simulink model "TransmissionController"  (R2023b)
settings: configuration reference "VehicleFixed10ms" (kept outside this file)
StartFcn:
  | %tic
StopFcn:
  | %toc
libraries: autolibtranscontrolscommon x1
settings Model: DataDictionary=VirtualVehicleTemplate.sldd  ModifiedByFormat=The MathWorks, Inc.  Creator=The MathWorks, Inc.  LastModifiedBy=The MathWorks, Inc.
settings ConfigSetRef: SourceName=VehicleFixed10ms

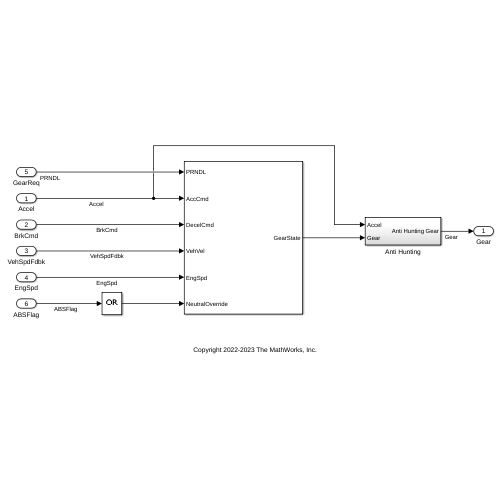
[thumbnail: Simulink's stored preview of the top-level diagram]
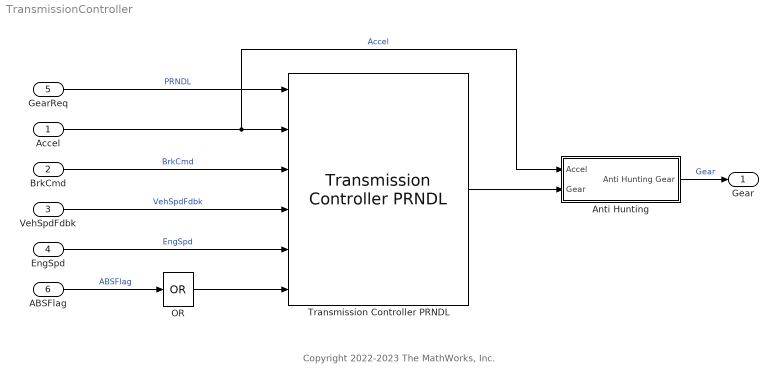
== system TransmissionController ==
  note: Copyright 2022-2023 The MathWorks, Inc.
  Accel : Inport  OutDataTypeStr=double  PortDimensions=1
  BrkCmd : Inport  Port=2  OutDataTypeStr=double  PortDimensions=1
  VehSpdFdbk : Inport  Port=3  OutDataTypeStr=double  Unit=m/s  PortDimensions=1
  EngSpd : Inport  Port=4  OutDataTypeStr=double  Unit=rad/s  PortDimensions=1
  GearReq : Inport  Port=5  OutDataTypeStr=double  PortDimensions=1
  ABSFlag : Inport  Port=6  OutDataTypeStr=boolean  PortDimensions=4
  Anti Hunting : Subsystem
  OR : Logic  Operator=OR  Inputs=1  AllPortsSameDT=off  OutDataTypeStr=boolean
  Transmission Controller PRNDL : autolibtranscontrolscommon/Transmission Controller PRNDL  DriveMode=off  GearInit=CtrlTcuInitGear  LugSpd=CtrlTcuLugSpd  MinUpSpd=CtrlTcuMinUpSpd  tClutchUp=CtrlTcuTmUpSh  tClutchDn=CtrlTcuTmDnSh  tPark=120  VelUnit=km/hr  UpShSpd=CtrlTcuUpShSpd  UpLdBpt=CtrlTcuUpLdBpt  UpShBpt=1:7  UpPtBpt=[1 2]  DnShfSpd=CtrlTcuDnShSpd  DnShSpd=CtrlTcuDnShSpd  DnLdBpt=CtrlTcuDnLdBpt  DnShBpt=2:8  DnPtBpt=[1 2]  POFS=zeros(4,1)  GOFS=zeros(1,7)  Ngears=8  aMode=6
  Gear : Outport  OutDataTypeStr=double  PortDimensions=1  VectorParamsAs1DForOutWhenUnconnected=off
  wires:
  ABSFlag/1 -> OR/1  "ABSFlag"
  Anti Hunting/1(Anti Hunting Gear) -> Gear/1  "Gear"
  GearReq/1 -> Transmission Controller PRNDL/1  "PRNDL"
  Accel/1 -> Anti Hunting/1(Accel), Transmission Controller PRNDL/2  "Accel"
  BrkCmd/1 -> Transmission Controller PRNDL/3  "BrkCmd"
  EngSpd/1 -> Transmission Controller PRNDL/5  "EngSpd"
  VehSpdFdbk/1 -> Transmission Controller PRNDL/4  "VehSpdFdbk"
  OR/1 -> Transmission Controller PRNDL/6
  Transmission Controller PRNDL/1 -> Anti Hunting/2(Gear)

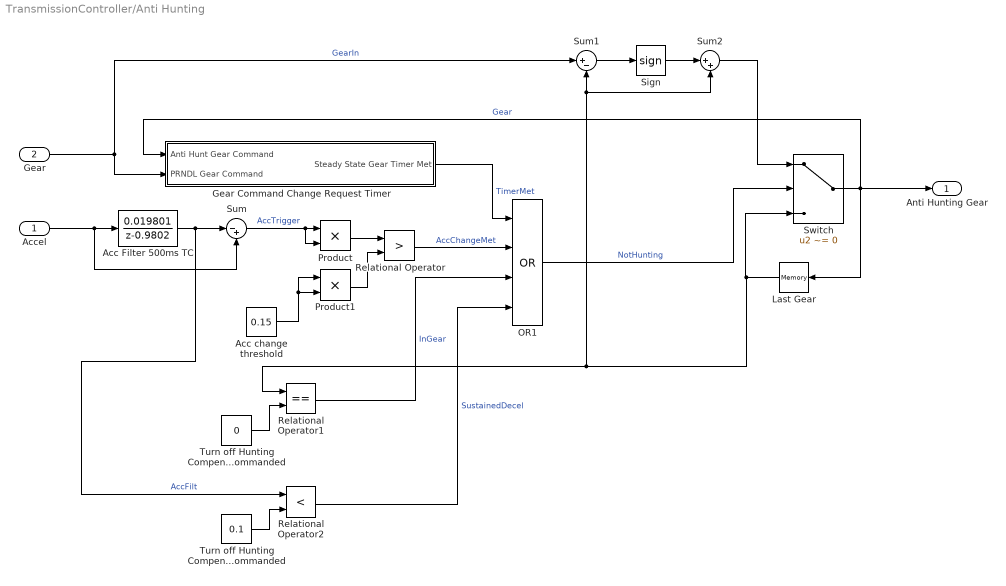
== system TransmissionController/Anti Hunting ==
  Accel : Inport
  Gear : Inport  Port=2
  Acc Filter 500ms TC : DiscreteTransferFcn  Numerator=[0,0.019801]  Denominator=[1,-0.9802]
  Acc change threshold : Constant  Value=0.15
  Gear Command Change Request Timer : Subsystem
  Last Gear : Memory  InheritSampleTime=on
  OR1 : Logic  Operator=OR  Inputs=4  IconShape=distinctive  AllPortsSameDT=off  OutDataTypeStr=boolean
  Product : Product
  Product1 : Product
  Relational Operator : RelationalOperator  Operator=>  OutDataTypeStr=boolean  RndMeth=Simplest  InputSameDT=off
  Relational Operator1 : RelationalOperator  Operator===  OutDataTypeStr=boolean  RndMeth=Simplest  InputSameDT=off
  Relational Operator2 : RelationalOperator  Operator=<  OutDataTypeStr=boolean  RndMeth=Simplest  InputSameDT=off
  Sign : Signum
  Sum : Sum  Inputs=|-+
  Sum1 : Sum  Inputs=|+-
  Sum2 : Sum  Inputs=|++
  Switch : Switch  Criteria=u2 ~= 0  SaturateOnIntegerOverflow=off  InputSameDT=off
  Turn off Hunting Compensation Sustained Decel Is Commanded : Constant  Value=0.1
  Turn off Hunting Compensation When Neutral Is Commanded : Constant  Value=0
  Anti Hunting Gear : Outport
  wires:
  Product1/1 -> Relational Operator/2
  Gear/1 -> Sum1/1, Gear Command Change Request Timer/2(PRNDL Gear Command)  "GearIn"
  Relational Operator/1 -> OR1/2  "AccChangeMet"
  Acc change threshold/1 -> Product1/1, Product1/2
  OR1/1 -> Switch/2  "NotHunting"
  Accel/1 -> Acc Filter 500ms TC/1, Sum/2
  Gear Command Change Request Timer/1(Steady State Gear Timer Met) -> OR1/1  "TimerMet"
  Sum/1 -> Product/2, Product/1  "AccTrigger"
  Last Gear/1 -> Relational Operator1/1, Sum2/2, Sum1/2, Switch/3
  Product/1 -> Relational Operator/1
  Acc Filter 500ms TC/1 -> Relational Operator2/1, Sum/1  "AccFilt"
  Turn off Hunting Compensation When Neutral Is Commanded/1 -> Relational Operator1/2
  Relational Operator1/1 -> OR1/3  "InGear"
  Turn off Hunting Compensation Sustained Decel Is Commanded/1 -> Relational Operator2/2
  Relational Operator2/1 -> OR1/4  "SustainedDecel"
  Switch/1 -> Gear Command Change Request Timer/1(Anti Hunt Gear Command), Anti Hunting Gear/1, Last Gear/1  "Gear"
  Sum1/1 -> Sign/1
  Sign/1 -> Sum2/1
  Sum2/1 -> Switch/1

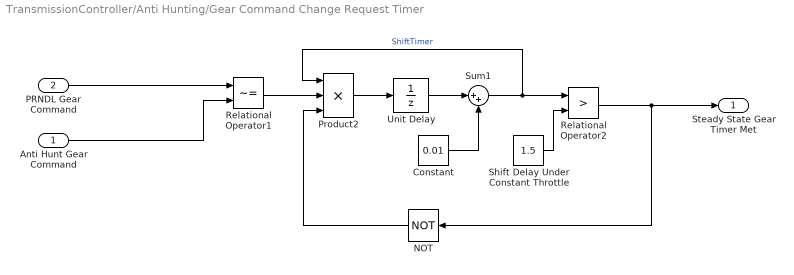
== system TransmissionController/Anti Hunting/Gear Command Change Request Timer ==
  Anti Hunt Gear Command : Inport
  PRNDL Gear Command : Inport  Port=2
  Constant : Constant  Value=0.01
  NOT : Logic  Operator=NOT  IconShape=distinctive  AllPortsSameDT=off  OutDataTypeStr=boolean
  Product2 : Product  Inputs=3
  Relational Operator1 : RelationalOperator  Operator=~=  OutDataTypeStr=boolean  RndMeth=Simplest  InputSameDT=off
  Relational Operator2 : RelationalOperator  Operator=>  OutDataTypeStr=boolean  RndMeth=Simplest  InputSameDT=off
  Shift Delay Under Constant Throttle : Constant  Value=1.5
  Sum1 : Sum  Inputs=|++
  Unit Delay : UnitDelay  SampleTime=-1  HasFrameUpgradeWarning=on
  Steady State Gear Timer Met : Outport
  wires:
  Unit Delay/1 -> Sum1/1
  Constant/1 -> Sum1/2
  Anti Hunt Gear Command/1 -> Relational Operator1/2
  Sum1/1 -> Product2/1, Relational Operator2/1  "ShiftTimer"
  PRNDL Gear Command/1 -> Relational Operator1/1
  Product2/1 -> Unit Delay/1
  Relational Operator2/1 -> NOT/1, Steady State Gear Timer Met/1
  Relational Operator1/1 -> Product2/2
  Shift Delay Under Constant Throttle/1 -> Relational Operator2/2
  NOT/1 -> Product2/3
